simulink model "PID_discreto"  (R2022b)
settings: Solver=VariableStepAuto  StartTime=0.0  StopTime=10.0  RelTol=1e-3
values from neighbouring files (symbols this model uses):
  Kd = Kp*Td    [get_PID.m]
  Ki = Kp/Ti    [get_PID.m]
  Kp = delta_k*cos(delta_phi)    [get_PID.m]
undefined symbols (not defined in the file or in its folder): A_step, aw_sw, DiscIntNeverNeededParam, Kw, PID_sw, sens, T, Tl
settings Model: Creator=marcoverri  LastModifiedBy=marcoverri

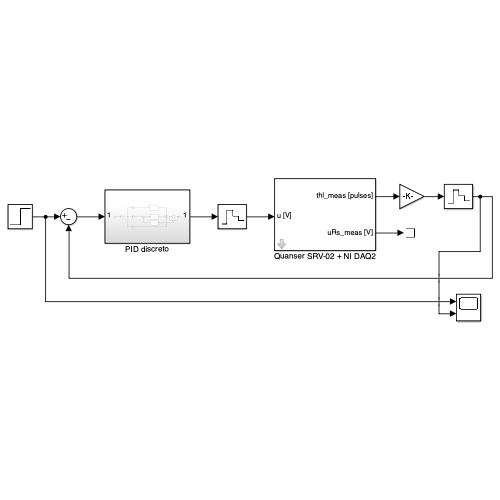
[thumbnail: Simulink's stored preview of the top-level diagram]
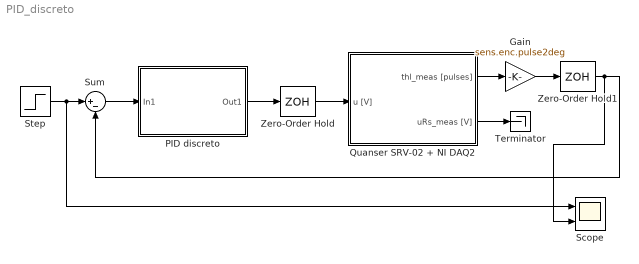
== system PID_discreto ==
  Gain : Gain  Gain=sens.enc.pulse2deg
  PID discreto : Subsystem
  Quanser SRV-02 + NI DAQ2 : Subsystem  mask(Quanser SRV-02 (with inertial load) + NI DAQ){Ts=0.001, fricType=Coulomb + viscous}
      mask prompts: Ts "NI DAQ Sample Time:"; fricType "Friction model"
      mask help: Quanser SRV-02 (with inertial load) + NI DAQ model.
      mask init:
      | %%  Sensors data
      | 
      | %   shunt resistor
      | sens.curr.Rs = 0.5;                         %   resistance [Ohm]   
      | sens.curr.uRs_std = 0.01;                   %   voltage noise standard dev [V]                           
      | sens.curr.uRs_var = sens.curr.uRs_std^2;	%   voltage noise variance [V^2]
      | 
      | %   Hewlett-Packard HEDS-5540#A06 optical encoder
      | sens.enc.ppr = 500*4;                       %   pulses per rotation
      | sens.enc.pulse2deg = 360/sens.enc.ppr;      %   [pulses] -> [deg]
      | sens.enc.pulse2rad = 2*pi/sens.enc.ppr;     %   [pulses] -> [rad]
      | sens.enc.deg2pulse = sens.enc.ppr/360;      %   [deg] -> [pulses]
      | sens.enc.rad2pulse = sens.enc.ppr/2/pi;     %   [rad] -> [pulses]
      | 
      | 
      | %%  Data acquisition board (daq) data
      | 
      | %   NI PCI-6221 DAC data
      | daq.dac.bits = 16;                                  %   resolution (bits)
      | daq.dac.fs   = 10;                                  %   full scale 
      | daq.dac.q    = 2*daq.dac.fs/(2^daq.dac.bits-1);     %	quantization
      | 
      | %   NI PCI-6221 ADC data
      | daq.adc.bits = 16;                                  %   resolution (bits)
      | daq.adc.fs   = 10;                                  %   full scale (as set in SLDRT Analog Input block)
      | daq.adc.q    = 2*daq.adc.fs/(2^daq.adc.bits-1);     %   quantization
      mask Help:
      | Riccardo Antonello (antonello@dei.unipd.it)
      | 
      | April 24, 2020
      | 
      | Dept. of Information Engineering, University of Padova
      mask TypeOptions fricType: Coulomb + viscous | Karnopp
  Scope : Scope  NumInputPorts=2
  Step : Step  After=A_step  SampleTime=0
  Sum : Sum  Inputs=|+-
  Terminator : Terminator
  Zero-Order Hold : ZeroOrderHold  SampleTime=T
  Zero-Order Hold1 : ZeroOrderHold  SampleTime=T
  wires:
  PID discreto/1(Out1) -> Zero-Order Hold/1
  Zero-Order Hold/1 -> Quanser SRV-02 + NI DAQ2/1(u [V])
  Quanser SRV-02 + NI DAQ2/1(thl_meas [pulses]) -> Gain/1
  Gain/1 -> Zero-Order Hold1/1
  Step/1 -> Scope/1, Sum/1
  Sum/1 -> PID discreto/1(In1)
  Zero-Order Hold1/1 -> Scope/2, Sum/2
  Quanser SRV-02 + NI DAQ2/2(uRs_meas [V]) -> Terminator/1

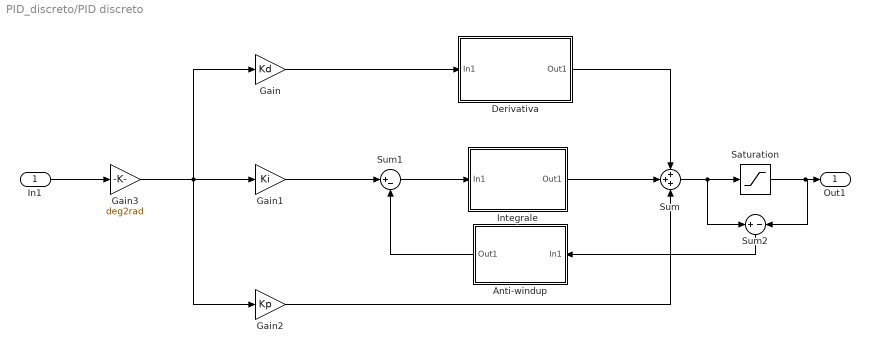
== system PID_discreto/PID discreto ==
  In1 : Inport
  Anti-windup : Subsystem
  Derivativa : Subsystem
  Gain : Gain  Gain=Kd
  Gain1 : Gain  Gain=Ki
  Gain2 : Gain  Gain=Kp
  Gain3 : Gain  Gain=deg2rad
  Integrale : Subsystem
  Saturation : Saturate  UpperLimit=12  LowerLimit=-12
  Sum : Sum  Inputs=+++
  Sum1 : Sum  Inputs=|+-
  Sum2 : Sum  Inputs=+|-
  Out1 : Outport
  wires:
  Gain2/1 -> Sum/3
  Sum/1 -> Saturation/1, Sum2/1
  In1/1 -> Gain3/1
  Gain3/1 -> Gain2/1, Gain/1, Gain1/1
  Saturation/1 -> Sum2/2, Out1/1
  Gain1/1 -> Sum1/1
  Sum1/1 -> Integrale/1(In1)
  Integrale/1(Out1) -> Sum/2
  Gain/1 -> Derivativa/1(In1)
  Derivativa/1(Out1) -> Sum/1
  Sum2/1 -> Anti-windup/1(In1)
  Anti-windup/1(Out1) -> Sum1/2

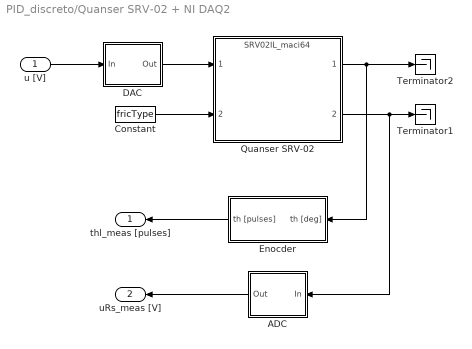
== system PID_discreto/Quanser SRV-02 + NI DAQ2 ==
  u [V] : Inport
  ADC : Subsystem
  Constant : Constant  Value=fricType
  DAC : Subsystem
  Enocder : Subsystem
  Quanser SRV-02 : ModelReference  ModelNameDialog=SRV02IL_maci64.slxp  ModelReferenceVersion=1.44  CopyOfModelProtected=on
  Terminator1 : Terminator
  Terminator2 : Terminator
  thl_meas [pulses] : Outport
  uRs_meas [V] : Outport  Port=2
  wires:
  Enocder/1(th [pulses]) -> thl_meas [pulses]/1
  ADC/1(Out) -> uRs_meas [V]/1
  DAC/1(Out) -> Quanser SRV-02/1
  Quanser SRV-02/2 -> ADC/1(In), Terminator1/1
  u [V]/1 -> DAC/1(In)
  Quanser SRV-02/1 -> Enocder/1(th [deg]), Terminator2/1
  Constant/1 -> Quanser SRV-02/2

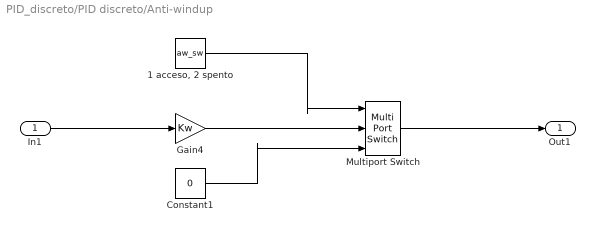
== system PID_discreto/PID discreto/Anti-windup ==
  In1 : Inport
  "1 acceso, 2 spento" : Constant  Value=aw_sw
  Constant1 : Constant  Value=0
  Gain4 : Gain  Gain=Kw
  Multiport Switch : MultiPortSwitch  Inputs=2  SaturateOnIntegerOverflow=off  InputSameDT=off
  Out1 : Outport
  wires:
  Multiport Switch/1 -> Out1/1
  In1/1 -> Gain4/1
  Gain4/1 -> Multiport Switch/2
  "1 acceso, 2 spento"/1 -> Multiport Switch/1
  Constant1/1 -> Multiport Switch/3

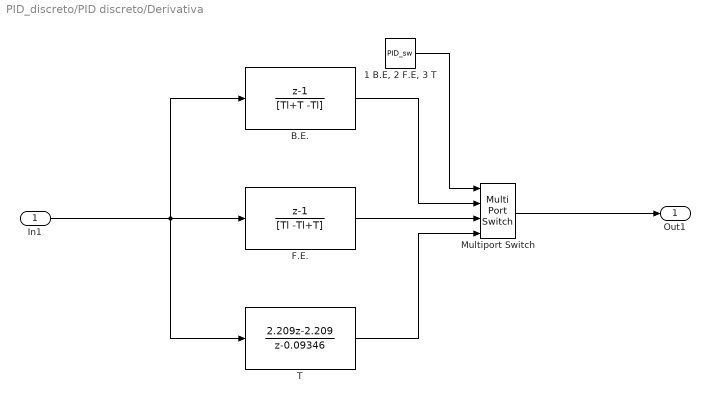
== system PID_discreto/PID discreto/Derivativa ==
  In1 : Inport
  "1 B.E, 2 F.E, 3 T" : Constant  Value=PID_sw
  B.E. : DiscreteTransferFcn  Numerator=[1 -1]  Denominator=[Tl+T -Tl]  SampleTime=T
  F.E. : DiscreteTransferFcn  Numerator=[1 -1]  Denominator=[Tl -Tl+T]  SampleTime=T
  Multiport Switch : MultiPortSwitch  SaturateOnIntegerOverflow=off  InputSameDT=off
  T : DiscreteTransferFcn  Numerator=[2.209 -2.209]  Denominator=[1 -0.09346]  SampleTime=T
  Out1 : Outport
  wires:
  Multiport Switch/1 -> Out1/1
  B.E./1 -> Multiport Switch/2
  F.E./1 -> Multiport Switch/3
  In1/1 -> T/1, F.E./1, B.E./1
  T/1 -> Multiport Switch/4
  "1 B.E, 2 F.E, 3 T"/1 -> Multiport Switch/1

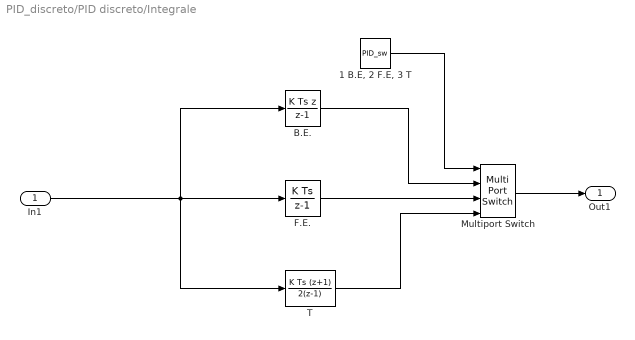
== system PID_discreto/PID discreto/Integrale ==
  In1 : Inport
  "1 B.E, 2 F.E, 3 T" : Constant  Value=PID_sw
  B.E. : DiscreteIntegrator  IntegratorMethod=Integration: Backward Euler  SampleTime=-1  ICPrevOutput=DiscIntNeverNeededParam  ICPrevScaledInput=DiscIntNeverNeededParam
  F.E. : DiscreteIntegrator  SampleTime=-1  ICPrevOutput=DiscIntNeverNeededParam  ICPrevScaledInput=DiscIntNeverNeededParam
  Multiport Switch : MultiPortSwitch  SaturateOnIntegerOverflow=off  InputSameDT=off
  T : DiscreteIntegrator  IntegratorMethod=Integration: Trapezoidal  SampleTime=-1  ICPrevOutput=DiscIntNeverNeededParam  ICPrevScaledInput=DiscIntNeverNeededParam
  Out1 : Outport
  wires:
  B.E./1 -> Multiport Switch/2
  F.E./1 -> Multiport Switch/3
  T/1 -> Multiport Switch/4
  Multiport Switch/1 -> Out1/1
  In1/1 -> T/1, F.E./1, B.E./1
  "1 B.E, 2 F.E, 3 T"/1 -> Multiport Switch/1

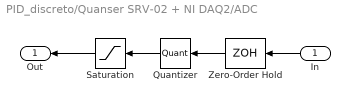
== system PID_discreto/Quanser SRV-02 + NI DAQ2/ADC ==
  In : Inport
  Quantizer : Quantizer  QuantizationInterval=daq.adc.q
  Saturation : Saturate  UpperLimit=daq.adc.fs  LowerLimit=-daq.adc.fs
  Zero-Order Hold : ZeroOrderHold  SampleTime=Ts
  Out : Outport
  wires:
  Saturation/1 -> Out/1
  In/1 -> Zero-Order Hold/1
  Quantizer/1 -> Saturation/1
  Zero-Order Hold/1 -> Quantizer/1

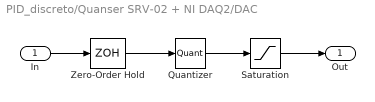
== system PID_discreto/Quanser SRV-02 + NI DAQ2/DAC ==
  In : Inport
  Quantizer : Quantizer  QuantizationInterval=daq.dac.q
  Saturation : Saturate  UpperLimit=daq.dac.fs  LowerLimit=-daq.dac.fs
  Zero-Order Hold : ZeroOrderHold  SampleTime=Ts
  Out : Outport
  wires:
  Quantizer/1 -> Saturation/1
  In/1 -> Zero-Order Hold/1
  Zero-Order Hold/1 -> Quantizer/1
  Saturation/1 -> Out/1

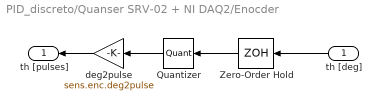
== system PID_discreto/Quanser SRV-02 + NI DAQ2/Enocder ==
  th [deg] : Inport
  Quantizer : Quantizer  QuantizationInterval=sens.enc.pulse2deg
  Zero-Order Hold : ZeroOrderHold  SampleTime=Ts
  deg2pulse : Gain  Gain=sens.enc.deg2pulse
  th [pulses] : Outport
  wires:
  Quantizer/1 -> deg2pulse/1
  th [deg]/1 -> Zero-Order Hold/1
  Zero-Order Hold/1 -> Quantizer/1
  deg2pulse/1 -> th [pulses]/1
